simulink model "vehicle_model_999"  (R2025b)
settings: Solver=ode23tb  StartTime=0.0  StopTime=50  MaxStep=0.001  RelTol=1e-3
values from neighbouring files (symbols this model uses):
  aero_par = struct()    [Load_aero_parameters.m]
  init_r = 0    [Run_this_first.m]
  init_vx = 0    [Run_this_first.m]
  init_vy = 0    [Run_this_first.m]
  m = Par.m    [LapSim_Endurance_final_ts_v2.m]    (also in Lap_Sim_Final_inverse.m = Par.Mass; Lapsim_Endurance_final_ts.m; New_LapSim_final_ts_v1.m = Par.Mass; Torque_vectoring_lookup_table_v3.m = 270)
  Par = struct()    [Load_vehicle_parameters.m]
  sus_par = struct()    [Load_sus_parameters.m]
  TireData = []    [Lapsim_final_for_app.m]
  V_ref = 45    [Run_this_first.m]
undefined symbols (not defined in the file or in its folder): Battery, Brake_Val, HP, Ki_data, Kp_data, Motor, steer_input, Steer_Val, TC_target_slip, Throttle_Val, vx_breakpoints
libraries: simulink x7, autolibshared x2, BatteryEstimators x1
(part 2 of 3)

== system vehicle_model_999/input_selector ==
  accln_sim : Inport
  for_maps : Inport  Port=2
  Saturation : Saturate  UpperLimit=1  LowerLimit=0
  Throttle Variant Subsystem : Subsystem  Variant=on
  throttle : Outport
  wires:
  Throttle Variant Subsystem/1(throttle) -> Saturation/1
  for_maps/1 -> Throttle Variant Subsystem/2(accln_input_for_map1)
  accln_sim/1 -> Throttle Variant Subsystem/1(accln)
  Saturation/1 -> throttle/1

== system vehicle_model_999/prevent_div_by_0 ==
  In1 : Inport
  Constant : Constant  Value=0.001
  Switch : Switch  Criteria=u2 > Threshold  SaturateOnIntegerOverflow=off  InputSameDT=off
  Out1 : Outport
  wires:
  In1/1 -> Switch/2, Switch/1
  Constant/1 -> Switch/3
  Switch/1 -> Out1/1

== system vehicle_model_999/prevent_div_by_1 ==
  In1 : Inport
  Constant : Constant  Value=0.001
  Switch : Switch  Criteria=u2 > Threshold  SaturateOnIntegerOverflow=off  InputSameDT=off
  Out1 : Outport
  wires:
  Switch/1 -> Out1/1
  Constant/1 -> Switch/3
  In1/1 -> Switch/1, Switch/2

== system vehicle_model_999/roll and pitch angles1 ==
  ax : Inport
  ay : Inport  Port=2
  F_aero : Inport  Port=3
  Phi_constants : MATLAB Function  TreatAsAtomicUnit=on
  Pitch : Subsystem
  Roll : Subsystem
  Scope : Scope  Commented=on  NumInputPorts=2
  theta_constants : MATLAB Function  TreatAsAtomicUnit=on
  phi : Outport
  Theta : Outport  Port=2
  wires:
  ax/1 -> Pitch/3(ax)
  Phi_constants/1(K_phi) -> Roll/1(K_phi)
  Phi_constants/2(C_phi) -> Roll/2(C_phi)
  ay/1 -> Roll/3(ay)
  Roll/1(phi) -> phi/1, Scope/2
  Pitch/1(Theta) -> Scope/1, Theta/1
  theta_constants/1(K_theta) -> Pitch/1(K_theta)
  theta_constants/2(C_theta) -> Pitch/2(C_theta)
  F_aero/1 -> Pitch/4(downforce)

== system vehicle_model_999/steer_input_simulink1 ==
  Ramp : simulink/Sources/Ramp  slope=pi/6  start=5  InitialOutput=0
  Out1 : Outport
  wires:
  Ramp/1 -> Out1/1

== system vehicle_model_999/throttle_input_simulink ==
  Clock : Clock
  Constant : Constant
  Constant1 : Constant  Value=0
  Saturation : Saturate  UpperLimit=1  LowerLimit=0
  Switch : Switch  Criteria=u2 > Threshold  Threshold=2  SaturateOnIntegerOverflow=off  InputSameDT=off
  accln_sim : Outport
  wires:
  Clock/1 -> Switch/2
  Switch/1 -> Saturation/1
  Constant1/1 -> Switch/1
  Constant/1 -> Switch/3
  Saturation/1 -> accln_sim/1

== system vehicle_model_999/visualise input ==
  InputBus : Inport
  Add : Sum
  Bus Creator : BusCreator  Inputs=4
  Bus Selector : BusSelector  OutputSignals=Torque_input,Steer_input
  Bus Selector1 : BusSelector  OutputSignals=T_rl,T_rr
  Demux : Demux
  Gain : Gain  Gain=180/pi
  Scope : Scope  NumInputPorts=3
      settings: ActiveDisplayYMinimum=-31.958230429629104  ActiveDisplayYMaximum=287.624073866662
  Terminator : Terminator
  Terminator1 : Terminator
  To Workspace : ToWorkspace  VariableName=Total_torque  SaveFormat=Timeseries  SampleTime=-1
  To Workspace1 : ToWorkspace  VariableName=Steering_deg  SaveFormat=Timeseries  SampleTime=-1
  wires:
  InputBus/1 -> Bus Selector/1
  Bus Selector/2 -> Gain/1, Scope/3  "<Steer_input>"
  Bus Selector/1 -> Demux/1  "<Torque_input>"
  Demux/1 -> Bus Creator/1
  Demux/2 -> Bus Creator/2
  Demux/3 -> Bus Creator/3  "T_rl"
  Demux/4 -> Bus Creator/4  "T_rr"
  Bus Creator/1 -> Bus Selector1/1
  Bus Selector1/1 -> Scope/1, Add/2  "<T_rl>"
  Bus Selector1/2 -> Scope/2, Add/1  "<T_rr>"
  Add/1 -> To Workspace/1, Terminator/1  "Total_torque"
  Gain/1 -> To Workspace1/1, Terminator1/1  "steering_deg"

== system vehicle_model_999/Camber1/Subsystem ==
  Camber : Inport
  Demux1 : Demux
  Gain : Gain  Gain=180/pi
  Scope : Scope  NumInputPorts=4
      settings: ActiveDisplayYMinimum=-0.50156  ActiveDisplayYMaximum=0.49315  DataLoggingVariableName=ScopeData17
  wires:
  Gain/1 -> Demux1/1
  Demux1/4 -> Scope/4  "RR"
  Demux1/3 -> Scope/3  "RL"
  Demux1/2 -> Scope/2  "FR"
  Demux1/1 -> Scope/1  "FL"
  Camber/1 -> Gain/1

== system vehicle_model_999/Camber1/Subsystem1 ==
  dynamic_camber : Inport
  Demux1 : Demux
  Gain : Gain  Gain=180/pi
  Scope : Scope  NumInputPorts=4
      settings: ActiveDisplayYMinimum=78.6694  ActiveDisplayYMaximum=79.6641  DataLoggingVariableName=ScopeData17
  wires:
  Gain/1 -> Demux1/1
  Demux1/4 -> Scope/4
  Demux1/3 -> Scope/3
  Demux1/2 -> Scope/2
  Demux1/1 -> Scope/1
  dynamic_camber/1 -> Gain/1

== system vehicle_model_999/Camber1/Subsystem2 ==
  static_camber : Inport
  Demux1 : Demux
  Gain : Gain  Gain=180/pi
  Scope : Scope  NumInputPorts=4
      settings: ActiveDisplayYMinimum=-1  ActiveDisplayYMaximum=1  DataLoggingVariableName=ScopeData17
  wires:
  static_camber/1 -> Gain/1
  Demux1/1 -> Scope/1
  Demux1/2 -> Scope/2
  Demux1/3 -> Scope/3
  Demux1/4 -> Scope/4
  Gain/1 -> Demux1/1

== system vehicle_model_999/Force and Torque Equilibrium/Subsystem ==
  In1 : Inport
  Clock : Clock
  Compare To Constant : simulink/Logic and Bit Operations/Compare To Constant  relop=>=  const=75  OutDataTypeStr=boolean
  Detect Rise Positive : simulink/Logic and Bit Operations/Detect Rise Positive  vinit=0  OutDataTypeStr=boolean
  Triggered Subsystem : Subsystem  TreatAsAtomicUnit=on
  Out1 : Outport
  wires:
  In1/1 -> Compare To Constant/1
  Detect Rise Positive/1 -> Triggered Subsystem/Trigger
  Clock/1 -> Triggered Subsystem/1(In1)
  Triggered Subsystem/1(Out1) -> Out1/1
  Compare To Constant/1 -> Detect Rise Positive/1

== system vehicle_model_999/Normal_loads1/ARB ==
  Zs : Inport
  MATLAB Function : MATLAB Function  TreatAsAtomicUnit=on
  Visualise F_arb : Subsystem  Commented=on
  F_arb : Outport
  wires:
  Zs/1 -> MATLAB Function/1(Zs)
  MATLAB Function/1(F_arb) -> Visualise F_arb/1(F_arb), F_arb/1

== system vehicle_model_999/Normal_loads1/Spring_forces ==
  theta : Inport
  phi : Inport  Port=2
  F_aero : Inport  Port=3
  MATLAB Function : MATLAB Function  TreatAsAtomicUnit=on
  Zs : Outport
  F_spring : Outport  Port=2
  Zs1 : Outport  Port=3
  wires:
  theta/1 -> MATLAB Function/1(theta)
  phi/1 -> MATLAB Function/2(phi)
  F_aero/1 -> MATLAB Function/3(F_aero_total)
  MATLAB Function/2(F_spring) -> F_spring/1
  MATLAB Function/1(Zs) -> Zs/1
  MATLAB Function/3(Zs1) -> Zs1/1

== system vehicle_model_999/Normal_loads1/Visualise F_spring ==
  F_spring : Inport
  Demux : Demux
  Scope : Scope  Commented=on  NumInputPorts=4
      settings: ActiveDisplayYMinimum=-696.9087  ActiveDisplayYMaximum=77.4343  DataLoggingVariableName=ScopeData26
  wires:
  Demux/1 -> Scope/1  "F_s_fl"
  Demux/2 -> Scope/2  "F_s_fr"
  Demux/3 -> Scope/3  "F_s_rl"
  Demux/4 -> Scope/4  "F_s_rr"
  F_spring/1 -> Demux/1

== system vehicle_model_999/Normal_loads1/Visualise Normal_Force ==
  F_z : Inport
  Demux : Demux
  Scope : Scope  NumInputPorts=4
      settings: ActiveDisplayYMinimum=585.93132450154008  ActiveDisplayYMaximum=755.3708910235755  DataLoggingVariableName=ScopeData26
  wires:
  Demux/4 -> Scope/4  "Fz_rr"
  Demux/3 -> Scope/3  "Fz_rl"
  Demux/2 -> Scope/2  "Fz_fr"
  Demux/1 -> Scope/1  "Fz_fl"
  F_z/1 -> Demux/1

== system vehicle_model_999/Normal_loads1/Visualise sus disp ==
  Zs : Inport
  Gain : Gain  Gain=-1000
  To Workspace : ToWorkspace  VariableName=zsfl  SaveFormat=Timeseries  SampleTime=-1
  To Workspace1 : ToWorkspace  VariableName=zsfr  SaveFormat=Timeseries  SampleTime=-1
  To Workspace2 : ToWorkspace  VariableName=zsrl  SaveFormat=Timeseries  SampleTime=-1
  To Workspace3 : ToWorkspace  VariableName=zsrr  SaveFormat=Timeseries  SampleTime=-1
  Zs in mm : MATLAB Function  TreatAsAtomicUnit=on
  Zs_in mm : Scope  Commented=on  NumInputPorts=4
      settings: ActiveDisplayYMinimum=-1  ActiveDisplayYMaximum=1  DataLoggingVariableName=ScopeData26
  wires:
  Zs/1 -> Gain/1
  Zs in mm/1(zsfl) -> Zs_in mm/1, To Workspace/1  "zsfl in mm"
  Zs in mm/2(zsfr) -> To Workspace1/1, Zs_in mm/2  "zsfr in mm"
  Zs in mm/3(zsrl) -> To Workspace2/1, Zs_in mm/3  "zsrl  in mm"
  Zs in mm/4(zsrr) -> To Workspace3/1, Zs_in mm/4  "zsrr in mm"
  Gain/1 -> Zs in mm/1(Zs)

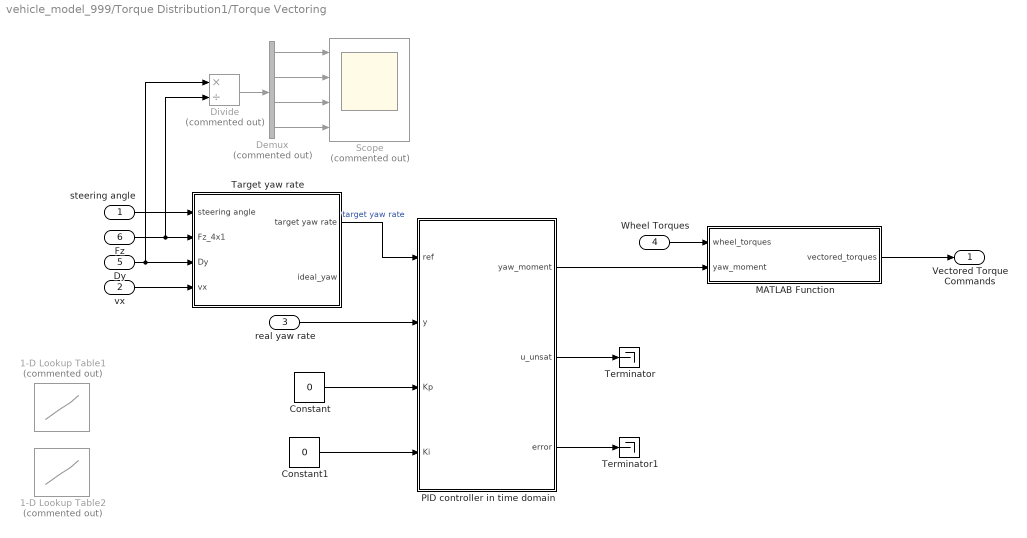
== system vehicle_model_999/Torque Distribution1/Torque Vectoring ==
  steering angle : Inport
  vx : Inport  Port=2
  real yaw rate : Inport  Port=3
  Wheel Torques : Inport  Port=4
  Dy : Inport  Port=5
  Fz : Inport  Port=6
  1-D Lookup Table1 : Lookup_n-D  Commented=on  NumberOfTableDimensions=1  BreakpointsForDimension1=vx_breakpoints  Table=Kp_data  InternalRulePriority=Speed  RndMeth=Simplest
  1-D Lookup Table2 : Lookup_n-D  Commented=on  NumberOfTableDimensions=1  BreakpointsForDimension1=vx_breakpoints  Table=Ki_data  InternalRulePriority=Speed  RndMeth=Simplest
  Constant : Constant  Value=0
  Constant1 : Constant  Value=0
  Demux : Demux  Commented=on
  Divide : Product  Commented=on  Inputs=*/
  MATLAB Function : MATLAB Function  TreatAsAtomicUnit=on
  PID controller in time domain : MATLAB Function  TreatAsAtomicUnit=on  SystemSampleTime=0.001
  Scope : Scope  Commented=on  NumInputPorts=4
      settings: ActiveDisplayYMinimum=-1  ActiveDisplayYMaximum=1  DataLoggingVariableName=ScopeData6
  Target yaw rate : Subsystem
  Terminator : Terminator
  Terminator1 : Terminator
  Vectored Torque Commands : Outport
  wires:
  steering angle/1 -> Target yaw rate/1(steering angle)
  Target yaw rate/1(target yaw rate) -> PID controller in time domain/1(ref)  "target yaw rate"
  Wheel Torques/1 -> MATLAB Function/1(wheel_torques)
  MATLAB Function/1(vectored_torques) -> Vectored Torque Commands/1
  vx/1 -> Target yaw rate/4(vx)
  Constant/1 -> PID controller in time domain/3(Kp)
  PID controller in time domain/1(yaw_moment) -> MATLAB Function/2(yaw_moment)
  Fz/1 -> Divide/2, Target yaw rate/2(Fz_4x1)
  Dy/1 -> Divide/1, Target yaw rate/3(Dy)
  Divide/1 -> Demux/1
  Demux/1 -> Scope/1
  Demux/2 -> Scope/2
  Demux/3 -> Scope/3
  Demux/4 -> Scope/4
  real yaw rate/1 -> PID controller in time domain/2(y)
  Constant1/1 -> PID controller in time domain/4(Ki)
  PID controller in time domain/2(u_unsat) -> Terminator/1
  PID controller in time domain/3(error) -> Terminator1/1

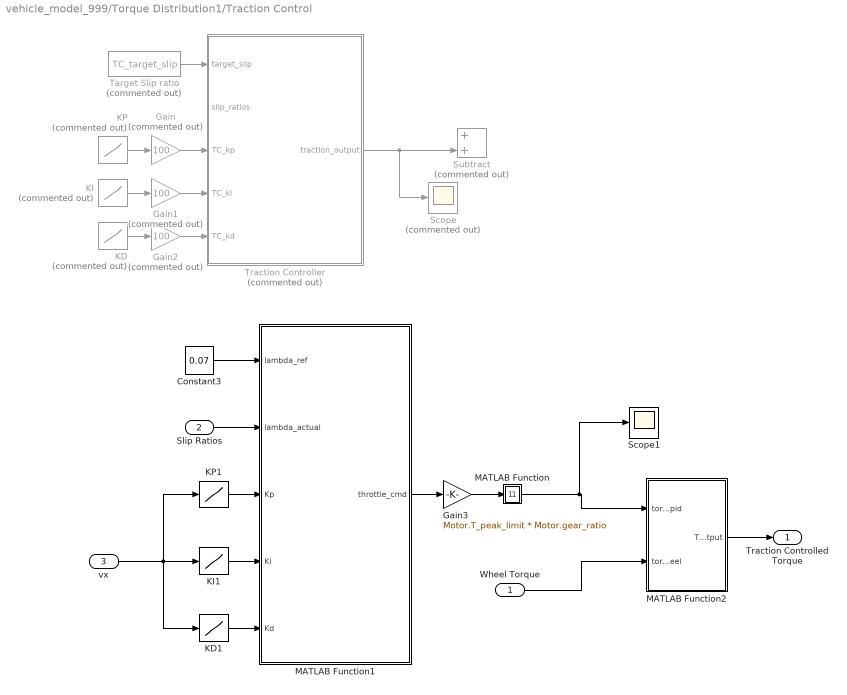
== system vehicle_model_999/Torque Distribution1/Traction Control ==
  Wheel Torque : Inport
  Slip Ratios : Inport  Port=2
  vx : Inport  Port=3
  Constant3 : Constant  Value=0.07
  Gain : Gain  Commented=on  Gain=100
  Gain1 : Gain  Commented=on  Gain=100
  Gain2 : Gain  Commented=on  Gain=100
  Gain3 : Gain  Gain=Motor.T_peak_limit * Motor.gear_ratio
  KD : Lookup_n-D  Commented=on  NumberOfTableDimensions=1  BreakpointsForDimension1=[0, 55e-10, 0.0045, 2, 8.5,9,100]  Table=[0, 0, 0.0014, 0.0109,0,0,0]  InternalRulePriority=Speed  RndMeth=Simplest
  KD1 : Lookup_n-D  NumberOfTableDimensions=1  BreakpointsForDimension1=[0, 55e-10, 0.0045, 2, 8.5,9]  Table=[0, 0, 0.0014, 0.0109,0,0]  InternalRulePriority=Speed  RndMeth=Simplest
  KI : Lookup_n-D  Commented=on  NumberOfTableDimensions=1  BreakpointsForDimension1=[0; 55e-10;0.0045; 2; 8.5;100]  Table=[0.1; 0.1;700; 500; 450;450 ]  InternalRulePriority=Speed  RndMeth=Simplest
  KI1 : Lookup_n-D  NumberOfTableDimensions=1  BreakpointsForDimension1=[0; 55e-10;0.0045; 2; 8.5]  Table=[0.1; 0.1;700; 500; 450 ]  InternalRulePriority=Speed  RndMeth=Simplest
  KP : Lookup_n-D  Commented=on  NumberOfTableDimensions=1  BreakpointsForDimension1=[0; 55e-10; 0.0045; 2; 8.5;100]  Table=[ 0.5; 0.5; 2.5; 10; 10;10]  InternalRulePriority=Speed  RndMeth=Simplest
  KP1 : Lookup_n-D  NumberOfTableDimensions=1  BreakpointsForDimension1=[0; 55e-10; 0.0045; 2; 8.5]  Table=[ 0.5; 0.5; 2.5; 10; 10]  InternalRulePriority=Speed  RndMeth=Simplest
  MATLAB Function : MATLAB Function  TreatAsAtomicUnit=on
  MATLAB Function1 : MATLAB Function  TreatAsAtomicUnit=on  SystemSampleTime=0.001
  MATLAB Function2 : MATLAB Function  TreatAsAtomicUnit=on
  Scope : Scope  Commented=on
      settings: ActiveDisplayYMinimum=-1  ActiveDisplayYMaximum=1  DataLoggingVariableName=ScopeData5
  Scope1 : Scope
      settings: ActiveDisplayYMinimum=-1  ActiveDisplayYMaximum=1  DataLoggingVariableName=ScopeData12
  Subtract : Sum  Commented=on
  Target Slip ratio : Constant  Commented=on  Value=TC_target_slip
  Traction Controller : MATLAB Function  Commented=on  TreatAsAtomicUnit=on
  Traction Controlled Torque : Outport
  wires:
  Traction Controller/1(traction_output) -> Scope/1, Subtract/2
  Target Slip ratio/1 -> Traction Controller/1(target_slip)
  KI/1 -> Gain1/1
  KP/1 -> Gain/1
  KD/1 -> Gain2/1
  Gain/1 -> Traction Controller/3(TC_kp)
  Gain1/1 -> Traction Controller/4(TC_ki)
  Gain2/1 -> Traction Controller/5(TC_kd)
  KD1/1 -> MATLAB Function1/5(Kd)
  MATLAB Function1/1(throttle_cmd) -> Gain3/1
  KI1/1 -> MATLAB Function1/4(Ki)
  KP1/1 -> MATLAB Function1/3(Kp)
  vx/1 -> KD1/1, KI1/1, KP1/1
  Slip Ratios/1 -> MATLAB Function1/2(lambda_actual)
  Constant3/1 -> MATLAB Function1/1(lambda_ref)
  Wheel Torque/1 -> MATLAB Function2/2(torque_wheel)
  Gain3/1 -> MATLAB Function/1(u)
  MATLAB Function/1(y) -> Scope1/1, MATLAB Function2/1(torque_pid)
  MATLAB Function2/1(TC_output) -> Traction Controlled Torque/1

== system vehicle_model_999/Torque Distribution1/is TCS on? ==
  traction_controlled_torque : Inport
  In1 : Inport  Port=2
  TV_T_wheel : Inport  Port=3
  Switch : Switch  Criteria=u2 > Threshold  SaturateOnIntegerOverflow=off  InputSameDT=off
  torque_output : Outport
  wires:
  In1/1 -> Switch/2
  Switch/1 -> torque_output/1
  TV_T_wheel/1 -> Switch/3
  traction_controlled_torque/1 -> Switch/1

== system vehicle_model_999/Torque Distribution1/is TV on? ==
  vectored_torque : Inport
  In1 : Inport  Port=2
  wheel_torque : Inport  Port=3
  Switch : Switch  Criteria=u2 > Threshold  SaturateOnIntegerOverflow=off  InputSameDT=off
  torque_output : Outport
  wires:
  wheel_torque/1 -> Switch/3
  vectored_torque/1 -> Switch/1
  Switch/1 -> torque_output/1
  In1/1 -> Switch/2

== system vehicle_model_999/input_select/Brake Variant Subsystem ==
  brake_sim : Inport
  vel : Inport  Port=2
  GGV : Subsystem  VariantControl=Mode_ggv
  Sideslip_vs_curvature_cst_accln : Subsystem  VariantControl=Mode_sideslip_vs_curvature_cst_accln
  Simulink : Subsystem  VariantControl=Mode_simulink
  curvature vs steer_angle : Subsystem  VariantControl=Mode_curvature_vs_steer
  sideslip_vs_curvature : Subsystem  VariantControl=Mode_sideslip_vs_curvature
  steerdiff_vs_ay : Subsystem  VariantControl=Mode_steerdiff_vs_ay
  timeseries : Subsystem  VariantControl=Mode_timeseries
  brake_input : Outport
  accln : Outport  Port=2

== system vehicle_model_999/input_selection/Steering Variant Subsystem ==
  In1 : Inport
  GGV : Subsystem  VariantControl=Mode_ggv
  Simulink : Subsystem  VariantControl=Mode_simulink
  Timeseries : Subsystem  VariantControl=Mode_timeseries
  curvature_vs_steering_angle : Subsystem  VariantControl=Mode_curvature_vs_steer
  sideslip_vs_curvature_1 : Subsystem  VariantControl=Mode_sideslip_vs_curvature
  sideslip_vs_curvature_constant_lat_accln : Subsystem  VariantControl=Mode_sideslip_vs_curvature_cst_accln
  steerdiff_vs_ay : Subsystem  VariantControl=Mode_steerdiff_vs_ay
  Steer Input : Outport

== system vehicle_model_999/input_selector/Throttle Variant Subsystem ==
  accln : Inport
  accln_input_for_map1 : Inport  Port=2
  GGV : Subsystem  VariantControl=Mode_ggv
  Simulink : Subsystem  VariantControl=Mode_simulink
  Timeseries : Subsystem  VariantControl=Mode_timeseries
  curvature vs steer : Subsystem  VariantControl=Mode_curvature_vs_steer
  sideslip_vs_curvature : Subsystem  VariantControl=Mode_sideslip_vs_curvature
  sideslip_vs_curvature_cst_accln : Subsystem  VariantControl=Mode_sideslip_vs_curvature_cst_accln
  steerdiff_vs_ay : Subsystem  VariantControl=Mode_steerdiff_vs_ay
  throttle : Outport

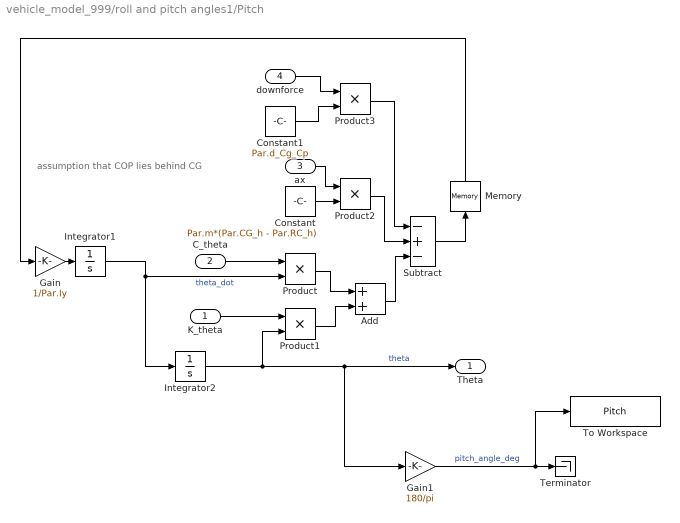
== system vehicle_model_999/roll and pitch angles1/Pitch ==
  note: assumption that COP lies behind CG
  K_theta : Inport
  C_theta : Inport  Port=2
  ax : Inport  Port=3
  downforce : Inport  Port=4
  Add : Sum
  Constant : Constant  Value=Par.m*(Par.CG_h - Par.RC_h)
  Constant1 : Constant  Value=Par.d_Cg_Cp
  Gain : Gain  Gain=1/Par.Iy
  Gain1 : Gain  Gain=180/pi
  Integrator1 : Integrator
  Integrator2 : Integrator
  Memory : Memory
  Product{,1..3} (4 alike) : Product
  Subtract : Sum  Inputs=-+-
  Terminator : Terminator
  To Workspace : ToWorkspace  VariableName=Pitch  SaveFormat=Timeseries  SampleTime=-1
  Theta : Outport
  wires:
  Gain/1 -> Integrator1/1
  Integrator1/1 -> Product/2, Integrator2/1  "theta_dot"
  C_theta/1 -> Product/1
  Integrator2/1 -> Theta/1, Gain1/1, Product1/2  "theta"
  K_theta/1 -> Product1/1
  Product/1 -> Add/1
  Product1/1 -> Add/2
  ax/1 -> Product2/1
  Constant/1 -> Product2/2
  Product2/1 -> Subtract/2
  Add/1 -> Subtract/3
  Subtract/1 -> Memory/1
  Memory/1 -> Gain/1
  downforce/1 -> Product3/1
  Constant1/1 -> Product3/2
  Product3/1 -> Subtract/1
  Gain1/1 -> To Workspace/1, Terminator/1  "pitch_angle_deg"

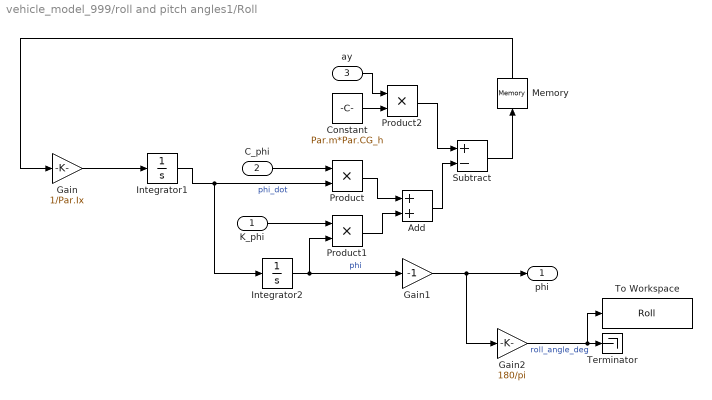
== system vehicle_model_999/roll and pitch angles1/Roll ==
  K_phi : Inport
  C_phi : Inport  Port=2
  ay : Inport  Port=3
  Add : Sum
  Constant : Constant  Value=Par.m*Par.CG_h
  Gain : Gain  Gain=1/Par.Ix
  Gain1 : Gain  Gain=-1
  Gain2 : Gain  Gain=180/pi
  Integrator1 : Integrator
  Integrator2 : Integrator
  Memory : Memory
  Product : Product
  Product1 : Product
  Product2 : Product
  Subtract : Sum  Inputs=+-
  Terminator : Terminator
  To Workspace : ToWorkspace  VariableName=Roll  SaveFormat=Timeseries  SampleTime=-1
  phi : Outport
  wires:
  Subtract/1 -> Memory/1
  Add/1 -> Subtract/2
  Product2/1 -> Subtract/1
  Constant/1 -> Product2/2
  ay/1 -> Product2/1
  Product1/1 -> Add/2
  Product/1 -> Add/1
  K_phi/1 -> Product1/1
  Integrator2/1 -> Gain1/1, Product1/2  "phi"
  C_phi/1 -> Product/1
  Integrator1/1 -> Integrator2/1, Product/2  "phi_dot"
  Gain/1 -> Integrator1/1
  Memory/1 -> Gain/1
  Gain2/1 -> To Workspace/1, Terminator/1  "roll_angle_deg"
  Gain1/1 -> Gain2/1, phi/1

== system vehicle_model_999/Force and Torque Equilibrium/Subsystem/Triggered Subsystem ==
  In1 : Inport
  Trigger : TriggerPort  VariantControl=(inherit)
  Out1 : Outport
  wires:
  In1/1 -> Out1/1

== system vehicle_model_999/Normal_loads1/ARB/Visualise F_arb ==
  F_arb : Inport
  Demux : Demux
  Scope : Scope  Commented=on  NumInputPorts=4
      settings: ActiveDisplayYMinimum=-1  ActiveDisplayYMaximum=1  DataLoggingVariableName=ScopeData11
  wires:
  F_arb/1 -> Demux/1
  Demux/1 -> Scope/1  "F_arb_fl"
  Demux/2 -> Scope/2  "F_arb_fr"
  Demux/3 -> Scope/3  "F_arb_rl"
  Demux/4 -> Scope/4  "F_arb_rr"

== system vehicle_model_999/Torque Distribution1/Torque Vectoring/Target yaw rate ==
  steering angle : Inport
  Fz_4x1 : Inport  Port=2
  Dy : Inport  Port=3
  vx : Inport  Port=4
  MATLAB Function : MATLAB Function  TreatAsAtomicUnit=on
  target yaw rate : Outport
  ideal_yaw : Outport  Port=2
  wires:
  vx/1 -> MATLAB Function/1(vx)
  Fz_4x1/1 -> MATLAB Function/4(Fz)
  Dy/1 -> MATLAB Function/3(Dy)
  steering angle/1 -> MATLAB Function/2(delta)
  MATLAB Function/1(target_yaw) -> target yaw rate/1
  MATLAB Function/2(ideal_yaw) -> ideal_yaw/1

== system vehicle_model_999/input_select/Brake Variant Subsystem/GGV ==
  Constant : Constant  Value=Brake_Val
  brake_input : Outport
  wires:
  Constant/1 -> brake_input/1

== system vehicle_model_999/input_select/Brake Variant Subsystem/Sideslip_vs_curvature_cst_accln ==
  vel : Inport
  Constant : Constant  Value=10
  Constant3 : Constant  Value=0
  Longitudinal Driver : autolibshared/Longitudinal Driver  extAccelOvr=off  extDecelOvr=off  extAccelHld=off  extDecelHld=off  extAccelZero=off  extDecelZero=off  cntrlType=PI  shftType=None  velUnits=m/s  gearOut=off  Kp=10  Ki=5  Kff=.1  Kg=0  VehVelVec=[0 100]  KffVec=[.1 .1]  KpVec=[10 10]  KiVec=[5 5]  KgVec=[0 0]  m=1500  Kpt=3000  tau=.1  L=2  aR=200  bR=2.5  cR=.5  g=9.81  vnom=5  Kaw=1  tauerr=.01  tauPt=2  GearInit=0  tShift=.1  pdlVec=[0.1 0.4 0.5 0.9]  upShftTbl=[-1 12.9375 26.4375 39.9375 51.18749999999999 62.4375 72.84375 83.25;-1 16.3125 29.8125 43.3125 54.5624 65.8125 76.78125 87.75;-1 19.6875 33.1875 46.68749999999999 57.9375 69.1875 80.71875 92.25;-1 33 52.5 77.25 100.5 138.75 161.875 185]  dwnShftTbl=[1 9.5625 23.0625 36.5625 47.8125 59.0625 68.90625 78.75;1 12.9375 26.4375 39.9375 51.18749999999999 62.4375 72.84375 83.25;1 16.3125 29.8125 43.3125 54.562499 65.8125 76.78125 87.75;1 19.6875 33.1875 46.68749999999999 57.9375 69.1875 80.71875 92.25]  tClutch=.5  tRev=.5  tPark=120  aMode=2  UpGearVec="[0  1  2  3  4  5  6  7]"  DownGearVec="[1  2  3  4  5  6  7  8]"
  Terminator1 : Terminator
  brake_input : Outport
  accln : Outport  Port=2
  wires:
  Constant3/1 -> Longitudinal Driver/3
  Constant/1 -> Longitudinal Driver/1
  Longitudinal Driver/1 -> Terminator1/1
  Longitudinal Driver/2 -> accln/1
  Longitudinal Driver/3 -> brake_input/1
  vel/1 -> Longitudinal Driver/2

== system vehicle_model_999/input_select/Brake Variant Subsystem/Simulink ==
  brake_sim : Inport
  brake_input : Outport
  wires:
  brake_sim/1 -> brake_input/1

== system vehicle_model_999/input_select/Brake Variant Subsystem/curvature vs steer_angle ==
  vel : Inport
  Constant : Constant  Value=V_ref
  Constant3 : Constant  Value=0
  Longitudinal Driver : autolibshared/Longitudinal Driver  extAccelOvr=off  extDecelOvr=off  extAccelHld=off  extDecelHld=off  extAccelZero=off  extDecelZero=off  cntrlType=PI  shftType=None  velUnits=m/s  gearOut=off  Kp=10  Ki=5  Kff=.1  Kg=0  VehVelVec=[0 100]  KffVec=[.1 .1]  KpVec=[10 10]  KiVec=[5 5]  KgVec=[0 0]  m=1500  Kpt=3000  tau=.1  L=2  aR=200  bR=2.5  cR=.5  g=9.81  vnom=5  Kaw=1  tauerr=.01  tauPt=2  GearInit=0  tShift=.1  pdlVec=[0.1 0.4 0.5 0.9]  upShftTbl=[-1 12.9375 26.4375 39.9375 51.18749999999999 62.4375 72.84375 83.25;-1 16.3125 29.8125 43.3125 54.5624 65.8125 76.78125 87.75;-1 19.6875 33.1875 46.68749999999999 57.9375 69.1875 80.71875 92.25;-1 33 52.5 77.25 100.5 138.75 161.875 185]  dwnShftTbl=[1 9.5625 23.0625 36.5625 47.8125 59.0625 68.90625 78.75;1 12.9375 26.4375 39.9375 51.18749999999999 62.4375 72.84375 83.25;1 16.3125 29.8125 43.3125 54.562499 65.8125 76.78125 87.75;1 19.6875 33.1875 46.68749999999999 57.9375 69.1875 80.71875 92.25]  tClutch=.5  tRev=.5  tPark=120  aMode=2  UpGearVec="[0  1  2  3  4  5  6  7]"  DownGearVec="[1  2  3  4  5  6  7  8]"
  Terminator : Terminator
  brake_input : Outport
  accln : Outport  Port=2
  wires:
  Longitudinal Driver/3 -> brake_input/1
  Constant3/1 -> Longitudinal Driver/3
  Longitudinal Driver/1 -> Terminator/1
  Constant/1 -> Longitudinal Driver/1
  Longitudinal Driver/2 -> accln/1
  vel/1 -> Longitudinal Driver/2

== system vehicle_model_999/input_select/Brake Variant Subsystem/sideslip_vs_curvature ==
  brake_sim : Inport
  brake_input : Outport
  wires:
  brake_sim/1 -> brake_input/1

== system vehicle_model_999/input_select/Brake Variant Subsystem/steerdiff_vs_ay ==
  Constant : Constant  Value=0
  brake_input : Outport
  wires:
  Constant/1 -> brake_input/1

== system vehicle_model_999/input_select/Brake Variant Subsystem/timeseries ==
  From Workspace : FromWorkspace  VariableName=brake_ts
  brake_input : Outport
  wires:
  From Workspace/1 -> brake_input/1

== system vehicle_model_999/input_selection/Steering Variant Subsystem/GGV ==
  SimInput_Steer : Constant  Value=Steer_Val
  Steer Input : Outport
  wires:
  SimInput_Steer/1 -> Steer Input/1

== system vehicle_model_999/input_selection/Steering Variant Subsystem/Simulink ==
  In1 : Inport
  Steer Input : Outport
  wires:
  In1/1 -> Steer Input/1

== system vehicle_model_999/input_selection/Steering Variant Subsystem/Timeseries ==
  From Workspace : FromWorkspace  VariableName=steer_ts
  Steer Input : Outport
  wires:
  From Workspace/1 -> Steer Input/1

== system vehicle_model_999/input_selection/Steering Variant Subsystem/curvature_vs_steering_angle ==
  Clock1 : Clock
  Constant1 : Constant  Value=0
  Ramp2 : simulink/Sources/Ramp  slope=pi/60  start=10  InitialOutput=0
  Saturation1 : Saturate  UpperLimit=pi/6
  Switch1 : Switch  Criteria=u2 > Threshold  Threshold=10  SaturateOnIntegerOverflow=off  InputSameDT=off
  Steer Input : Outport
  wires:
  Switch1/1 -> Saturation1/1
  Ramp2/1 -> Switch1/1
  Clock1/1 -> Switch1/2
  Constant1/1 -> Switch1/3
  Saturation1/1 -> Steer Input/1

== system vehicle_model_999/input_selection/Steering Variant Subsystem/sideslip_vs_curvature_1 ==
  Clock : Clock
  Constant : Constant  Value=0
  Constant1 : Constant  Value=steer_input
  Saturation : Saturate  UpperLimit=pi/20
  Switch : Switch  Criteria=u2 > Threshold  Threshold=4  SaturateOnIntegerOverflow=off  InputSameDT=off
  Steer Input : Outport
  wires:
  Switch/1 -> Saturation/1
  Saturation/1 -> Steer Input/1
  Constant1/1 -> Switch/1
  Clock/1 -> Switch/2
  Constant/1 -> Switch/3

== system vehicle_model_999/input_selection/Steering Variant Subsystem/sideslip_vs_curvature_constant_lat_accln ==
  Clock : Clock
  Constant : Constant  Value=0
  Ramp : simulink/Sources/Ramp  slope=pi/100  start=4  InitialOutput=0
  Saturation : Saturate  UpperLimit=pi/20
  Switch : Switch  Criteria=u2 > Threshold  Threshold=4  SaturateOnIntegerOverflow=off  InputSameDT=off
  Steer Input : Outport
  wires:
  Switch/1 -> Saturation/1
  Saturation/1 -> Steer Input/1
  Ramp/1 -> Switch/1
  Clock/1 -> Switch/2
  Constant/1 -> Switch/3

== system vehicle_model_999/input_selection/Steering Variant Subsystem/steerdiff_vs_ay ==
  Clock : Clock
  Constant : Constant  Value=0
  Ramp : simulink/Sources/Ramp  slope=pi/30  start=5  InitialOutput=0
  Saturation : Saturate  UpperLimit=pi/6  LowerLimit=0
  Switch : Switch  Criteria=u2 > Threshold  Threshold=5  SaturateOnIntegerOverflow=off  InputSameDT=off
  Steer Input : Outport
  wires:
  Switch/1 -> Saturation/1
  Ramp/1 -> Switch/1
  Constant/1 -> Switch/3
  Clock/1 -> Switch/2
  Saturation/1 -> Steer Input/1

== system vehicle_model_999/input_selector/Throttle Variant Subsystem/GGV ==
  SimInput_Throttle : Constant  Value=Throttle_Val
  throttle : Outport
  wires:
  SimInput_Throttle/1 -> throttle/1

== system vehicle_model_999/input_selector/Throttle Variant Subsystem/Simulink ==
  accln : Inport
  throttle : Outport
  wires:
  accln/1 -> throttle/1

== system vehicle_model_999/input_selector/Throttle Variant Subsystem/Timeseries ==
  From Workspace : FromWorkspace  VariableName=throttle_ts
  throttle : Outport
  wires:
  From Workspace/1 -> throttle/1

== system vehicle_model_999/input_selector/Throttle Variant Subsystem/curvature vs steer ==
  accln_input_for_map1 : Inport
  throttle : Outport
  wires:
  accln_input_for_map1/1 -> throttle/1

== system vehicle_model_999/input_selector/Throttle Variant Subsystem/sideslip_vs_curvature ==
  Constant : Constant
  throttle : Outport
  wires:
  Constant/1 -> throttle/1

== system vehicle_model_999/input_selector/Throttle Variant Subsystem/sideslip_vs_curvature_cst_accln ==
  accln_input_for_map1 : Inport
  throttle : Outport
  wires:
  accln_input_for_map1/1 -> throttle/1

== system vehicle_model_999/input_selector/Throttle Variant Subsystem/steerdiff_vs_ay ==
  Clock : Clock
  Constant1 : Constant  Value=0.25
  Ramp : simulink/Sources/Ramp  slope=2  start=0  InitialOutput=0
  Saturation : Saturate  UpperLimit=1  LowerLimit=0
  Switch : Switch  Criteria=u2 > Threshold  Threshold=4  SaturateOnIntegerOverflow=off  InputSameDT=off
  throttle : Outport
  wires:
  Clock/1 -> Switch/2
  Ramp/1 -> Switch/3
  Switch/1 -> Saturation/1
  Constant1/1 -> Switch/1
  Saturation/1 -> throttle/1

== matlab function vehicle_model_999/Rolling Resistance ==
  data: Fz input; wFx_rr output; Omega input; slip_angles input; Par parameter
function wFx_rr  = fcn(Fz, Omega,slip_angles, Par)
%#codegen

    % 1. Calculate Total Magnitude
    F_mag = Par.C_rr .* abs(Fz);

    % 2. Determine Direction
    Dir = tanh(10 * Omega);

    
    % X-Component: Resists Spin (Torque generating)
    % wFx = -Magnitude * Direction * cos(Alpha)
    wFx_rr = -F_mag .*Dir.* cos(slip_angles);

end

== matlab function vehicle_model_999/Rolling and Drag forces/Rolling Forces ==
  data: Fz input; Fx_rr_b output; Steer_FL input; Steer_FR input; Fy_rr_b output; Par parameter
function [Fx_rr_b, Fy_rr_b] = fcn(Fz, Steer_FL, Steer_FR, Par)

    %#codegen

    % 1. Setup
    C_rr = Par.C_rr; 
    
    % Construct Steering Vector (Assuming Rear Steer = 0)
    Delta = [Steer_FL; Steer_FR; 0; 0];

    % Initialize Outputs
    Fx_rr_b = zeros(4, 1);
    Fy_rr_b = zeros(4, 1);

    % 2. Calculate & Resolve Forces (Vectorized Loop)
    for i = 1:4
        
        % Magnitude (Always positive Fz)
        F_mag = C_rr * abs(Fz(i));
        
        % B. Define Force Vector in Wheel Frame
        F_xw = - F_mag;
        F_yw = 0;
        
        % C. Transform to Body Frame (Rotation)
        d = Delta(i);
        c = cos(d);
        s = sin(d);
        
        % Rotate: F_body = Rz(delta) * F_wheel
        % Fx_b = Fx_w*cos - Fy_w*sin
        Fx_rr_b(i) = F_xw * c - F_yw * s;
        
        % Fy_b = Fx_w*sin + Fy_w*cos
        Fy_rr_b(i) = F_xw * s + F_yw * c;
    end

end

== matlab function vehicle_model_999/Force and Torque Equilibrium/Force and Torque Equilibrium ==
  data: B_Fx input; ax output size=1; ay output size=1; B_Fy input; B_Fx_roll input; B_Fy_roll input; B_F_drag input; yawrate input; vx input; vy input; r_dot output size=1; Par parameter; ay_sensor output; ax_sensor output
function [ax, ay, r_dot,ay_sensor,ax_sensor] = fcn(B_Fx, B_Fy, B_Fx_roll, B_Fy_roll, B_F_drag, yawrate, vx, vy, Par)
%#codegen

    % 1. Enforce Column Vectors 
    % (Protects against dimension mismatch if an input is accidentally 1x4)
    B_Fx = B_Fx(:);
    B_Fy = B_Fy(:);
    B_Fx_roll = B_Fx_roll(:);
    B_Fy_roll = B_Fy_roll(:);

    % 2. Geometry Setup
    m = Par.m;
    Iz = Par.Iz;
    
    % Create Geometry Vectors for [FL; FR; RL; RR]
    % x_arms: Distance from CG to axle (Positive = Front)
    x_arms = [Par.Lf;   Par.Lf;  -Par.Lr;  -Par.Lr];
    
    % y_arms: Distance from centerline (Positive = Left)
    t = Par.TW / 2;
    y_arms = [-t;      t;       -t;      t];

    % 3. Total Corner Forces
    Fx_total = B_Fx + B_Fx_roll; 
    Fy_total = B_Fy + B_Fy_roll; 
    
    % 4. Linear Force Equilibrium
    Sigma_Fx = sum(Fx_total) - B_F_drag(1);
    Sigma_Fy = sum(Fy_total) - B_F_drag(2);
    
    % 5. Linear Accelerations 
    ax = (Sigma_Fx / m) + (vy * yawrate);
    ay = (Sigma_Fy / m) - (vx * yawrate);
    ay_sensor = Sigma_Fy/m;
    ax_sensor = Sigma_Fx/m;
    % 6. Moment Equilibrium (Vectorized)
    % Mz = (x * Fy) - (y * Fx)
    % We use .* for element-wise multiplication across all 4 wheels at once
    Mz_individual = (x_arms .* Fy_total) - (y_arms .* Fx_total);
    
    Sigma_Mz = sum(Mz_individual);
    
    % 7. Yaw Acceleration (rad/s^2)
    r_dot = Sigma_Mz / Iz;
end

== matlab function vehicle_model_999/Rolling and Drag forces/Aero Drag ==
  data: vx input; B_F_aero output; vy input; aero_par parameter
function B_F_aero = fcn(vx, vy, aero_par)

    %#codegen
    % AERODYNAMIC DRAG (Body Frame)
    % Calculates drag vector acting on the CG.
%
% Inputs:
%   vx, vy : Vehicle Velocities in Body Frame [m/s]
%   Par    : Parameters (.Cd, .Area, .rho, .C_side)
%
% Output:
%   B_F_aero : [Fx; Fy; 0] Aerodynamic Force Vector [N]

    % 1. Longitudinal Drag (Standard)
    % Fx = -0.5 * rho * Cd * Area * vx^2
    % Usage: sign(vx) ensures drag always opposes motion
    Fx_drag = 0.5 * aero_par.rho * aero_par.Cd * aero_par.Area * vx * abs(vx);

    % 2. Lateral Drag (Side Force) - Optional
    % Only relevant if sliding significantly.
    % If Par.C_side is not defined, calculate as 0.
    if isfield(aero_par, 'C_side') && aero_par.C_side > 0
        % Side area is often approx same as Frontal Area or larger
        % Fy = - 0.5 * rho * C_side * Area_Side * vy^2
        Fy_drag = -0.5 * aero_par.rho * aero_par.C_side * aero_par.Area * vy * abs(vy);
    else
        Fy_drag = 0;
    end
    
    % 3. Output Vector for Equilibrium Block
    B_F_aero = [Fx_drag; Fy_drag; 0];

end

== matlab function vehicle_model_999/Torque Distribution1/MATLAB Function ==
  data: T_wheel input; omega input; T_FL output; T_brake_vec input; T_FR output; T_RL output; T_RR output
function [T_FL, T_FR, T_RL, T_RR] = torque_combiner(T_wheel, omega, T_brake_vec)
    % INPUTS:
    % T_motor:     2x1 [Left, Right] Motor Torque Request (from Throttle)
    % omega:       4x1 [FL, FR, RL, RR] Wheel Speeds (rad/s)
    % T_brake_vec: 4x1 Brake Capacity (Negative values expected)

    % --- 1. INITIALIZATION ---
    T_FL = 0.0; T_FR = 0.0; T_RL = 0.0; T_RR = 0.0;
    
    % PARAMETERS
    w_threshold = 2.0;  % [rad/s] Speed below which we switch to linear damping
    brake_active_threshold = 100.0; % [Nm] Torque to consider "Brakes Active"

    % Get absolute brake capacities
    B_FL = abs(T_brake_vec(1));
    B_FR = abs(T_brake_vec(2));
    B_RL = abs(T_brake_vec(3));
    B_RR = abs(T_brake_vec(4));

    % --- 2. BRAKE PRIORITY LOGIC (The Fix for Rear Spin) ---
    % If the driver is braking hard, we CUT or REDUCE motor torque.
    % This prevents the "fighting" that causes the rear wheels to spin at 115 rad/s.
    
    total_brake_force = B_FL + B_FR + B_RL + B_RR;
    
    % Factor: 1.0 = Full Drive, 0.0 = Throttle Cut
    % If braking > threshold, we smoothly cut throttle to 0.
    if total_brake_force > brake_active_threshold
        throttle_factor = 0.0; 
    else
        throttle_factor = 1.0;
    end
    
    % Apply the cut to the motor inputs
    T_motor_effective = T_wheel * throttle_factor;


    % --- 3. ROBUST BRAKE CALCULATION (Viscous Region) ---
    % This local logic prevents solver crashes when wheels lock (w=0)
    % It uses linear damping near zero speed.
    
    % Fronts (Brake Only)
    T_FL = apply_brake_physics(omega(1), B_FL, w_threshold);
    T_FR = apply_brake_physics(omega(2), B_FR, w_threshold);

    % Rears (Motor + Brake)
    T_brake_RL = apply_brake_physics(omega(3), B_RL, w_threshold);
    T_brake_RR = apply_brake_physics(omega(4), B_RR, w_threshold);
    
    % Combine: Effective Motor (Positive) + Braking (Negative)
    T_RL = T_motor_effective(3) + T_brake_RL;
    T_RR = T_motor_effective(4) + T_brake_RR;
end

% --- HELPER LOGIC ---
function T_out = apply_brake_physics(w, Capacity, w_th)
    % If moving fast: Constant Friction (Capacity)
    % If moving slow: Viscous Damping (Linear line to 0)
    if abs(w) < w_th
        % Linear region (Like moving through honey)
        % This forces the torque to exactly 0 as speed hits 0.
        T_out = -Capacity * (w / w_th);
    else
        % Sliding region (Full friction)
        T_out = -Capacity * sign(w);
    end
end

== matlab function vehicle_model_999/Torque Distribution1/Torque Vectoring/MATLAB Function ==
  data: vectored_torques output; wheel_torques input; yaw_moment input; Par parameter; Motor parameter
function vectored_torques = fcn(wheel_torques,yaw_moment,Par,Motor)
max_wheel_torque = Motor.T_peak_limit * Motor.gear_ratio* Motor.overall_efficiency;
torque_difference = yaw_moment*(Par.R0/(Par.TW));
T_FL = wheel_torques(1);    
T_FR = wheel_torques(2);
T_RL = max(0,min(wheel_torques(3) - (torque_difference/2),max_wheel_torque));
T_RR = max(0,min(wheel_torques(4) + (torque_difference/2),max_wheel_torque));

vectored_torques = [T_FL; T_FR; T_RL; T_RR];

== matlab function vehicle_model_999/Torque Distribution1/Torque Vectoring/PID controller in time domain ==
  settings: updateMethod=DISCRETE
  data: ref input; yaw_moment output; y input; Kp input; Ki input; Par parameter; u_unsat output; error output; Motor parameter
function [yaw_moment,u_unsat,error] = pid_controller(ref, y, Kp, Ki,Par,Motor)
T = Par.TW;
R0 = Par.R0;
Half_T = T/2;


% Custom PI Controller with Clamping Anti-Windup

% Motor torque limits
T_max_motor = Motor.T_peak_limit*Motor.gear_ratio*Motor.overall_efficiency;  
T_min_motor = 0;  

% Force limit of each tire:
f_max = T_max_motor/R0;
f_min = T_min_motor/R0;

% Yaw_moment limits
u_max = f_max * Half_T;
u_min = f_min * Half_T;

% Persistent variables
persistent integral prev_error;
if isempty(integral)
    integral = 0;
    prev_error = 0;
end

% Sample time
T = 0.001;

% Compute error
error = ref - y;

% **Proportional Term**
P = Kp * error;

% **Integral Term with Clamping**
I = Ki * integral;

% Compute raw control signal
u_unsat = P + I;

%Clamping Anti-Windup
if u_unsat > u_max
    yaw_moment = u_max;
    % Freeze integral
elseif u_unsat < u_min
    yaw_moment = u_min;
    % Freeze integral
else
    yaw_moment = u_unsat;
    % Update integral only if NOT saturated
    integral = integral + 0.5* T * (error + prev_error);
end

% Store previous error
prev_error = error;
end

== matlab function vehicle_model_999/Torque Distribution1/Torque Vectoring/Target yaw rate/MATLAB Function ==
  data: vx input; target_yaw output; delta input; Dy input; Fz input; Par parameter; ideal_yaw output
function  [target_yaw,ideal_yaw]= target_yaw_rate(vx,delta,Dy,Fz,Par)

    ku = (Par.Lr*Par.m/(35238.459*(Par.Lf+Par.Lr))) - (Par.Lf*Par.m/(35033.582*(Par.Lf+Par.Lr)));   %understeer gradient
    epsilon = 0.01;                                                                                 %prevent division by zero
    ideal_yaw = delta*vx/(((vx+epsilon)^2*ku)+(Par.Lf+Par.Lr));                                     %from Ackermann formula

    if delta > deg2rad(1) || delta < -deg2rad(8) && vx > 3
        
        epsilon = 0.01;                                                                             %prevent division by zero
        
        mu_4x1 = Dy./Fz;                                                                            %from tire formula
        avg_mu = mean(mu_4x1(3:4));   % RL RR (if order = [FL FR RL RR])
        mu_4x1 = avg_mu;   
        
        yaw_limit = mu_4x1*Par.g/(vx + epsilon);                                                    %accounting grip limits
        
        if ideal_yaw < - yaw_limit 
            target_yaw = - yaw_limit;
        elseif ideal_yaw > yaw_limit
            target_yaw = yaw_limit;
        else 
            target_yaw = ideal_yaw;
        end
    else
    target_yaw = 0;
    end
end

== matlab function vehicle_model_999/Camber/MATLAB Function ==
  data: gamma_FR output; ay input; gamma_FL output; gamma_RL output; gamma_RR output; delta input; Par parameter; sus_par parameter
function [gamma_FR,gamma_FL,gamma_RL,gamma_RR] = fcn(ay,delta,Par, sus_par)

%% Static camber
gamma_static_f = sus_par.Camber_static;
gamma_static_r = sus_par.Camber_static;
% track_width = par.TW;
%% SUSPENSION ROLL STIFFNESS
k_phi1 = sus_par.Ks_f;  % front axle roll stiffness (Nm/rad)
k_phi2 = sus_par.Ks_r;  % rear axle roll stiffness (Nm/rad)

%% ROLL CENTER HEIGHTS
q1 = sus_par.RC_h_f;      % front roll center height (m)
q2 = sus_par.RC_h_r;      % rear roll center height (m)

%% CAMBER GEOMETRY
b1 = sus_par.IC_y_f;       % front IC horizontal distance (m)
b2 = sus_par.IC_y_r;       % rear IC horizontal distance (m)

%% TOTAL ROLL STIFFNESS
k_phi_total = k_phi1 + k_phi2;

%% TOTAL VEHICLE ROLL ANGLE
phi = Par.m.*ay.*Par.CG_h / k_phi_total;   % rad

%% AXLE ROLL ANGLES
phi_s1 = phi * (k_phi1 / k_phi_total);   % front suspension roll
phi_s2 = phi * (k_phi2 / k_phi_total);   % rear suspension roll

%% CAMBER GAIN COEFFICIENTS
k_gamma_f = - (q1 - b1) / b1;   % front
k_gamma_r = - (q2 - b2) / b2;   % rear

%% Camber due to roll on front axle
delta_gamma_roll_f = k_gamma_f * phi_s1;

%% Camber due to roll on rear axle
delta_gamma_roll_r = k_gamma_r * phi_s2;

%% Camber gain due to heave
% delta_gamma_heave_f = atan(Zwc_f/par.L_fvsa);
% delta_gamma_heave_r = atan(Zwc_r/par.L_fvsa);

%% Camber due to caster 
delta_gamma_caster = atan(tan(sus_par.Caster_static).*sin(delta));

%% Camber angle
gamma_FL = gamma_static_f + delta_gamma_roll_f + delta_gamma_caster;
gamma_FR = gamma_static_f - (delta_gamma_roll_f + delta_gamma_caster);
gamma_RL = gamma_static_r + delta_gamma_roll_r + delta_gamma_caster;
gamma_RR = gamma_static_r - (delta_gamma_roll_r + delta_gamma_caster);
end

== matlab function vehicle_model_999/Rolling and Drag forces/MATLAB Function ==
  data: u input; y output
function y = fcn(u)

y = u(1);

== matlab function vehicle_model_999/Torque Distribution1/Traction Control/MATLAB Function1 ==
  settings: updateMethod=DISCRETE
  data: lambda_ref input; lambda_actual input size=[4 1]; throttle_cmd output; Kp input; Ki input; Kd input
function throttle_cmd = pid_traction_controller(lambda_ref, lambda_actual, ...
Kp, Ki, Kd)
%#codegen

dt = 0.001;

persistent integrator prev_error;

if isempty(integrator)
    integrator = 0;
end

if isempty(prev_error)
    prev_error = 0;
end

    % ── Error ───────────────────────────────────────
    e = lambda_ref - lambda_actual(3);

    % ── Derivative (rate of slip change) ────────────
    de = (e - prev_error) / dt;

    % ── Conditional Integration (ANTI-WINDUP) ───────
    if abs(e) < 0.2   % integrate only near target
        integrator = integrator + e * dt;
    end

    integrator = max(min(integrator, 0.5), -0.5);

    % ── PID Output ──────────────────────────────────
    throttle_pid = Kp * e + Ki * integrator + Kd * de;

    % ── Clamp output ────────────────────────────────
    throttle_pid = max(min(throttle_pid, 1.0), 0.0);

    % ── Traction control logic ──────────────────────
    throttle_cmd = throttle_pid;

    % ── Store previous error ────────────────────────
    prev_error = e;


end

== matlab function vehicle_model_999/Torque Distribution1/Traction Control/MATLAB Function ==
  data: u input; y output
function y = fcn(u)
y = zeros(4,1);
y(3) = u;
y(4) = u;

== matlab function vehicle_model_999/Battery Pack/MATLAB Function ==
  data: Voc_pack input; v_bus output; R0_pack input; V_rc input; I_dc input
function v_bus = fcn(Voc_pack, R0_pack, V_rc, I_dc)
    % This function calculates the terminal voltage of the battery pack.
    % Voc_pack: Output from OCV LUT multiplied by Ns
    % R0_pack:  Output from R0 LUT multiplied by (Ns/Np)
    % V_rc:     Instantaneous voltage across the RC branch
    % I_dc:     Total DC current from the motor

    % 1. Calculate the instantaneous Ohmic drop (Ohm's Law)
    V_ohmic = I_dc * R0_pack;

    % 2. Calculate terminal voltage (Vt = Voc - V_ohmic - V_rc)
    v_bus = Voc_pack - V_ohmic - V_rc;

    % 3. Safety: Ensure voltage doesn't drop below a physical floor (e.g., 2.5V * Ns)
    % This prevents simulation crashes if the battery is fully depleted.
    v_bus = max(v_bus, 2.5 * 144); 
end

== matlab function vehicle_model_999/Brakes/MATLAB Function ==
  data: brake_pedal input; T_brakes output; omega input; Brake parameter; T_mag_Front output; T_mag_Rear output
function [T_brakes,T_mag_Front,T_mag_Rear]  = fcn(brake_pedal, omega, Brake)
    % BRAKE TORQUE CALCULATION
    % Converts normalized pedal/actuator position into physical torque
    % and ensures torque direction opposes wheel rotation.
    
    % 1. Calculate Magnitude of Torque based on Command (0-1)
    % We use the static max targets from the design sheet
    T_mag_Front = brake_pedal * Brake.MaxTorque_Wheel_F;
    T_mag_Rear  = brake_pedal * Brake.MaxTorque_Wheel_R;
    
    % Initialize output vector (FL, FR, RL, RR)
    T_brakes = zeros(4, 1);
    
    % 2. Apply Torque per Wheel with Directional Logic
    % Loop through all 4 wheels to apply logic individually
    % Indices: 1=FL, 2=FR, 3=RL, 4=RR
    
    for i = 1:4
        % Determine if this is a Front (1,2) or Rear (3,4) wheel
        if i <= 2
            T_req = T_mag_Front;
        else
            T_req = T_mag_Rear;
        end
        
        % Directional Check:
        % Torque must be negative if omega is positive, and vice versa.
        % -sign(omega) flips the torque direction.
        T_applied = T_req * -sign(omega(i));
        
        % Zero-Speed Cutoff:
        % If wheel is nearly stopped, clamp torque to zero to prevent 
        % the simulation from "driving" the car backwards.
        % if abs(omega(i)) < Brake.ZeroSpeedThreshold
        %     T_applied = 0;
        % 
            % Advanced: Ideally, below threshold, T_brake should act as 
            % a viscous damper or Coulomb friction that exactly cancels 
            % remaining motion, but zeroing is sufficient for laptime sims.
        % end
        
        T_brakes(i) = T_applied;
    end
end

== matlab function vehicle_model_999/Motor/Motor with Field Weakening ==
  data: rpm_4x1 input; Torque_Nm_vec output; throttle_scalar input; v_dc_bus input; Motor parameter; I_dc_total output size=[1]; P_total_sum output size=[1]
function [Torque_Nm_vec, I_dc_total,P_total_sum] = fcn(rpm_4x1, throttle_scalar, v_dc_bus, Motor)
    % Inputs:
    %   rpm_4x1         : [FL; FR; RL; RR] wheel speeds in RPM
    %   throttle_scalar : Driver input (0 to 1)
    %   v_dc_bus        : Battery voltage (V)
    %   Motor           : Struct containing constants
    
    % --- 1. Distribute Inputs ---
    % We apply the same throttle to both motors for now.
    % We extract the Rear-Left (index 3) and Rear-Right (index 4) speeds.
    rpm_targets = [rpm_4x1(3); rpm_4x1(4)]; 
    throttle_vec = [throttle_scalar; throttle_scalar];

    % Initialize storage
    Torque_Nm_vec = zeros(2, 1); % [T_RL; T_RR]
    P_elec_vec = zeros(2, 1);
    
    for i = 1:2
        % --- 2. Redline & Mechanical Limit Check ---
        if abs(rpm_targets(i)) >= Motor.n_max
            continue; % Torque and Power remain 0
        end

        % --- 3. Electrical Conversions ---
        omega_m = rpm_targets(i) * (2*pi/60);
        omega_e = max(abs(omega_m * Motor.p), 0.1); 
        V_max_phase = v_dc_bus / sqrt(3);
        I_cmd_peak = Motor.I_max_rms * sqrt(2) * throttle_vec(i);

        % --- 4. Region Selection: MTPA vs Field Weakening ---
        V_req_mtpa = omega_e * sqrt((Motor.L * I_cmd_peak)^2 + Motor.psi_m^2);
        
        if V_req_mtpa <= V_max_phase
            id = 0;
            iq = I_cmd_peak;
        else
            % Field Weakening logic for Fischer Motor
            a = Motor.L^2;
            b = 2 * Motor.L * Motor.psi_m;
            c = Motor.psi_m^2 + (Motor.L * I_cmd_peak)^2 - (V_max_phase / omega_e)^2;
            
            id = (-b + sqrt(max(0, b^2 - 4 * a * c))) / (2 * a);
            id = max(min(id, 0), -I_cmd_peak); 
            iq = sqrt(max(0, I_cmd_peak^2 - id^2));
        end

        % --- 5. Torque and Power Calculation ---
        T_gen = 1.5 * Motor.p * Motor.psi_m * iq;
        Torque_Nm_vec(i) = min(T_gen, Motor.T_peak_limit);

        % P_elec = P_mechanical + P_copper_losses
        P_mech = abs(Torque_Nm_vec(i) * omega_m);
        P_copper = 3 * 0.126 * (I_cmd_peak / sqrt(2))^2;
        P_elec_vec(i) = P_mech + P_copper;
    end

    % --- 6. Battery Summation ---
    P_total_sum = sum(P_elec_vec);
    if v_dc_bus > 20
        % Calculate total current draw for the Molicel P45B pack
        I_dc_total = P_total_sum / (0.95 * v_dc_bus);

    else
        I_dc_total = 0;
    end
end

== matlab function vehicle_model_999/Torque Distribution1/Traction Control/MATLAB Function2 ==
  data: TC_output output; torque_pid input; torque_wheel input
function TC_output = fcn(torque_pid, torque_wheel)
% Initialize TC_output
TC_output = zeros(4,1);

for i = 1:4

    if torque_pid(i) < torque_wheel(i)
        TC_output(i) = torque_pid(i);
    else
        TC_output(i) = torque_wheel(i);
    end
end
